simulink model "Copy_of_FIR"  (R2020b)
settings: Solver=FixedStepAuto  StartTime=0.0  StopTime=10.0  FixedStep=0.2  RelTol=1e-3
settings Model: Creator=DELL  LastModifiedBy=DELL
settings DataIOCC: SaveOutput=off  SaveTime=off

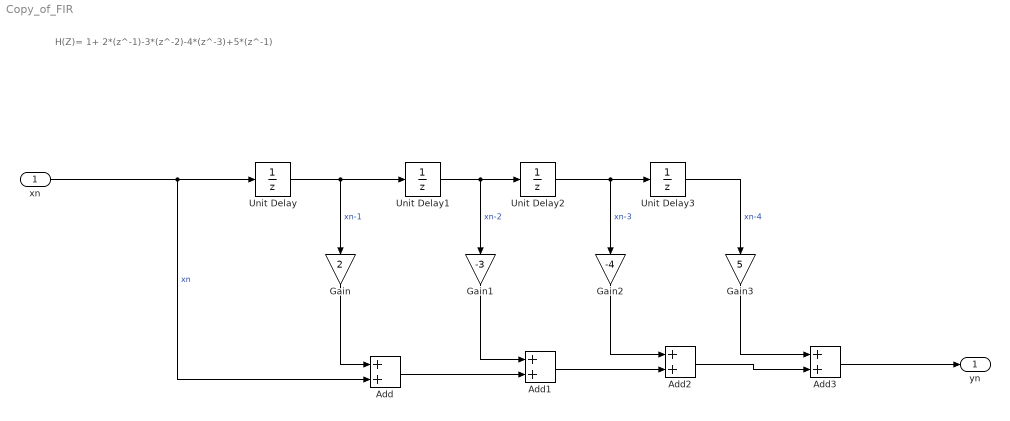
== system Copy_of_FIR ==
  note: H(Z)= 1+ 2*(z^-1)-3*(z^-2)-4*(z^-3)+5*(z^-1)
  xn : Inport  OutDataTypeStr=double  PortDimensions=1  SampleTime=[0.20000000000000001,0]
  Add{,1..3} (4 alike) : Sum
  Gain : Gain  Gain=2
  Gain1 : Gain  Gain=-3
  Gain2 : Gain  Gain=-4
  Gain3 : Gain  Gain=5
  Unit Delay{,1..3} (4 alike) : UnitDelay  SampleTime=-1  HasFrameUpgradeWarning=on
  yn : Outport  OutDataTypeStr=double  PortDimensions=1  SampleTime=[0.20000000000000001,0]
  wires:
  Unit Delay/1 -> Unit Delay1/1, Gain/1  "xn-1"
  Gain3/1 -> Add3/1
  Unit Delay1/1 -> Unit Delay2/1, Gain1/1  "xn-2"
  Unit Delay3/1 -> Gain3/1  "xn-4"
  Gain/1 -> Add/1
  Add/1 -> Add1/2
  xn/1 -> Unit Delay/1, Add/2  "xn"
  Add2/1 -> Add3/2
  Unit Delay2/1 -> Unit Delay3/1, Gain2/1  "xn-3"
  Add1/1 -> Add2/2
  Gain1/1 -> Add1/1
  Gain2/1 -> Add2/1
  Add3/1 -> yn/1
